simulink model "heights_linear"  (R2022b)
settings: Solver=VariableStepAuto  StartTime=0.0  StopTime=10  RelTol=1e-3
values from neighbouring files (symbols this model uses):
  U = 3:10    [ASTANK2_tasks.m]
undefined symbols (not defined in the file or in its folder): A, A_test, B, B_test, C, C_test, D, D_test
settings Model: Creator=Mucmu  LastModifiedBy=Mucmu

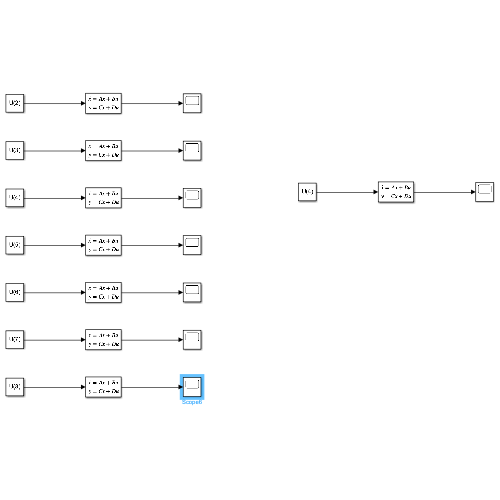
[thumbnail: Simulink's stored preview of the top-level diagram]
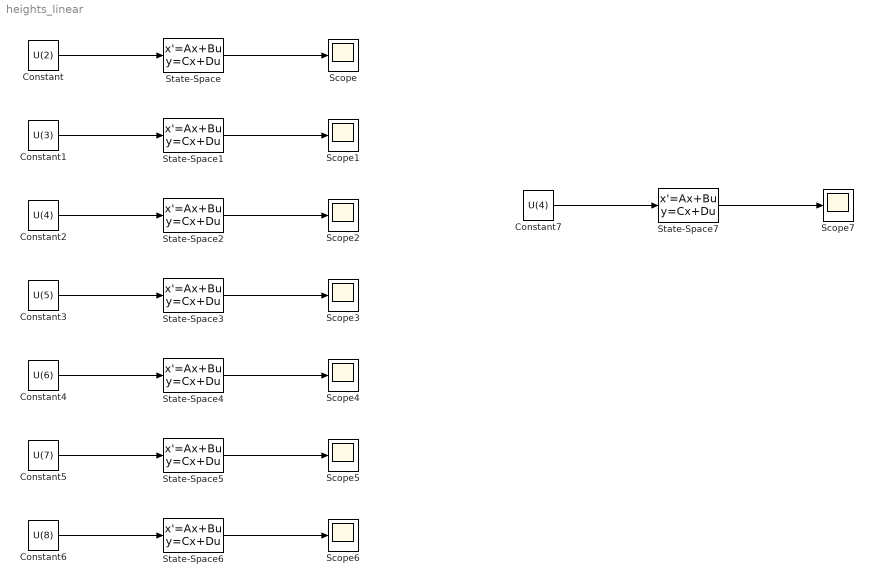
== system heights_linear ==
  Constant : Constant  Value=U(2)
  Constant1 : Constant  Value=U(3)
  Constant2 : Constant  Value=U(4)
  Constant3 : Constant  Value=U(5)
  Constant4 : Constant  Value=U(6)
  Constant5 : Constant  Value=U(7)
  Constant6 : Constant  Value=U(8)
  Constant7 : Constant  Value=U(4)
  Scope{,1..7} (8 alike) : Scope
  State-Space : StateSpace  A=A(:, :, 2)  B=B(:, :, 2)  C=C(:, :, 2)  D=D(:, :, 2)  InitialCondition=0
  State-Space1 : StateSpace  A=A(:, :, 3)  B=B(:, :, 3)  C=C(:, :, 3)  D=D(:, :, 3)  InitialCondition=0
  State-Space2 : StateSpace  A=A(:, :, 4)  B=B(:, :, 4)  C=C(:, :, 4)  D=D(:, :, 4)  InitialCondition=0
  State-Space3 : StateSpace  A=A(:, :, 5)  B=B(:, :, 5)  C=C(:, :, 5)  D=D(:, :, 5)  InitialCondition=0
  State-Space4 : StateSpace  A=A(:, :, 6)  B=B(:, :, 6)  C=C(:, :, 6)  D=D(:, :, 6)  InitialCondition=0
  State-Space5 : StateSpace  A=A(:, :, 7)  B=B(:, :, 7)  C=C(:, :, 7)  D=D(:, :, 7)  InitialCondition=0
  State-Space6 : StateSpace  A=A(:, :, 8)  B=B(:, :, 8)  C=C(:, :, 8)  D=D(:, :, 8)  InitialCondition=0
  State-Space7 : StateSpace  A=A_test  B=B_test  C=C_test  D=D_test  InitialCondition=0
  wires:
  Constant/1 -> State-Space/1
  State-Space/1 -> Scope/1
  State-Space1/1 -> Scope1/1
  Constant1/1 -> State-Space1/1
  State-Space2/1 -> Scope2/1
  Constant2/1 -> State-Space2/1
  State-Space3/1 -> Scope3/1
  Constant3/1 -> State-Space3/1
  State-Space4/1 -> Scope4/1
  Constant6/1 -> State-Space6/1
  State-Space6/1 -> Scope6/1
  State-Space5/1 -> Scope5/1
  Constant5/1 -> State-Space5/1
  Constant4/1 -> State-Space4/1
  Constant7/1 -> State-Space7/1
  State-Space7/1 -> Scope7/1
